simulink model "PI_real_expe"  (R2018a)
settings: Solver=FixedStepAuto  StartTime=0.0  StopTime=40  RelTol=1e-3
PreLoadFcn:
  | % plant
  | K0=0.82;
  | tau0=0.26;
  | 
  | % Sampling time
  | Ts=0.01;
  | 
  | % Especifications
  | xi=1;
  | ts_2=0.8; % settling time with %2 criterion
  | Tdes=ts_2/4;
  | wn=5.8/(xi*ts_2);
  | 
  | % Controller design
  | Zdes=exp(-Ts/Tdes);
  | alpha=exp(-Ts/tau0);
  | beta=-2*exp(-Ts*xi*wn)*cos(wn*Ts*sqrt(1-xi^2));
  | gamma=exp(-2*Ts*xi*wn);
  | 
  | Ki_star=(gamma-alpha+beta+(alpha+1))/(2*K0*(1-alpha));
  | Ki=(2/Ts)*Ki_star;
  | Kp=((beta+alpha+1)/(K0*(1-alpha)))-Ki_star;
undefined symbols (not defined in the file or in its folder): DiscIntNeverNeededParam
libraries: arduinolib x4, simulink x1
settings Model: SimulationMode=external  ExtModeTrigDuration=2  Creator=Eneko Lerma  LastModifiedBy=Eneko Lerma
settings OptimizationCC: EnhancedBackFolding=on  PassReuseOutputArgsAs=Individual arguments  MaxStackSize=64  OptimizeBlockOrder=speed  DifferentSizesBufferReuse=on  OptimizationCustomize=off
settings DebuggingCC: ParameterPrecisionLossMsg=none  ParameterTunabilityLossMsg=error
settings HardwareCC: ProdBitPerPointer=32  ProdBitPerSizeT=32  ProdBitPerPtrDiffT=32  ProdLargestAtomicInteger=Long  ProdLargestAtomicFloat=Double  ProdWordSize=32  ProdHWDeviceType=ARM Compatible->ARM Cortex
settings SFSimCC: MATLABDynamicMemAlloc=off
settings RTWCC: SystemTargetFile=ert.tlc  HardwareBoard=Arduino Due  TLCOptions=-aInlineSetEventsForThisBaseRateFcn=TLC_FALSE -aSuppressMultiTaskScheduler=TLC_FALSE -aRateBasedStepFcn=1  TemplateMakefile=ert_default_tmf  GenerateReport=on  Toolchain=Arduino ARM  BuildConfiguration=Faster Runs  IncludeHyperlinkInReport=on  LaunchReport=on  GenerateTraceInfo=on  GenerateTraceReport=on  GenerateTraceReportSl=on  GenerateTraceReportSf=on  GenerateTraceReportEml=on
settings RTWCC: CustomTerminator=|
  | writeDigitalPin((uint8_T)3, 0);
  | writeDigitalPin((uint8_T)5, 0);
settings CodeAppCC: ForceParamTrailComments=on  IgnoreCustomStorageClasses=off  OperatorAnnotations=on  SimulinkDataObjDesc=on  SFDataObjDesc=on  InsertBlockDesc=on
settings ERTTargetCC: SupportContinuousTime=on  SupportVariableSizeSignals=on

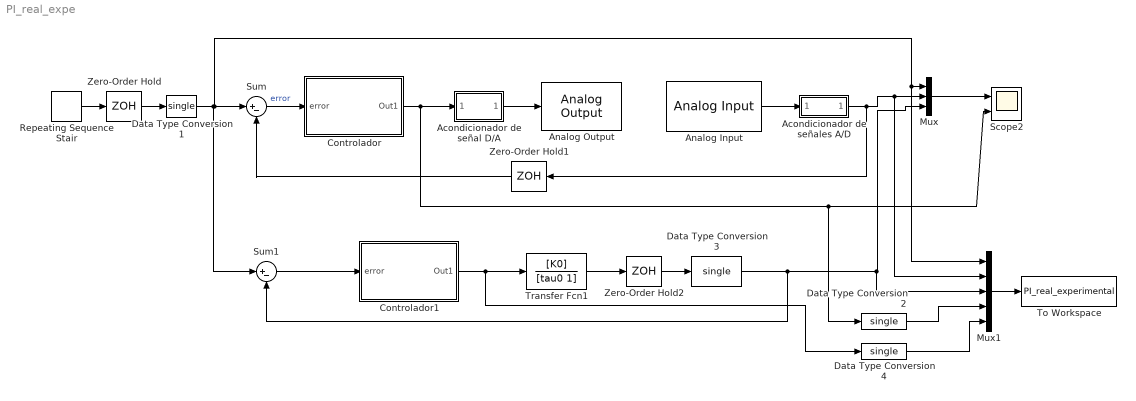
== system PI_real_expe ==
  Acondicionador de señal D/A : Subsystem
  Acondicionador de señales A/D : Subsystem
  Analog Input : arduinolib/Analog Input  pinNumber=0  ReadResultsOnly=off  ConversionTriggerSource=Software  ExternalTriggerType=uint32(0)  OutputDataType=uint16  EnableConversionCompleteNotify=off  EnableOuputStatus=off  SampleTime=0.005  blockPlatform=arduino
  Analog Output : arduinolib/Analog Output  DACpin=DAC1  blockPlatform=arduino
      settings: SourceProductName=Simulink Support Package for Arduino Hardware  SourceProductBaseCode=ARDUINO
  Controlador : Subsystem
  Controlador1 : Subsystem
  Data Type Conversion{1..4} (4 alike) : DataTypeConversion  OutDataTypeStr=single
  Mux : Mux  Inputs=3
  Mux1 : Mux  Inputs=5
  Repeating Sequence Stair : simulink/Sources/Repeating Sequence Stair  OutValues=[0 2 -2 -1].'  tsamp=4  OutMin=[]  OutMax=[]  OutDataTypeStr=double  OutputDataTypeScalingMode=double  OutDataType=fixdt(0,8)  ConRadixGroup=Best Precision: Vector-wise  OutScaling=2^-12
  Scope2 : Scope  NumInputPorts=2
  Sum : Sum  Inputs=|+-  AccumDataTypeStr=single
  Sum1 : Sum  Inputs=|+-  AccumDataTypeStr=single
  To Workspace : ToWorkspace  VariableName=PI_real_experimental  SaveFormat=Structure With Time  SampleTime=-1
  Transfer Fcn1 : TransferFcn  Numerator=[K0]  Denominator=[tau0 1]
  Zero-Order Hold : ZeroOrderHold  SampleTime=Ts
  Zero-Order Hold1 : ZeroOrderHold  SampleTime=Ts
  Zero-Order Hold2 : ZeroOrderHold  SampleTime=Ts
  wires:
  Mux/1 -> Scope2/1
  Acondicionador de señales A/D/1(" ") -> Mux1/2, Mux/2, Zero-Order Hold1/1
  Data Type Conversion1/1 -> Sum1/1, Sum/1, Mux1/1, Mux/1
  Sum/1 -> Controlador/1(error)  "error"
  Acondicionador de señal D/A/1(" ") -> Analog Output/1
  Analog Input/1 -> Acondicionador de señales A/D/1("  ")
  Controlador/1(Out1) -> Data Type Conversion2/1, Scope2/2, Acondicionador de señal D/A/1("  ")
  Zero-Order Hold/1 -> Data Type Conversion1/1
  Zero-Order Hold1/1 -> Sum/2
  Controlador1/1(Out1) -> Data Type Conversion4/1, Transfer Fcn1/1
  Sum1/1 -> Controlador1/1(error)
  Transfer Fcn1/1 -> Zero-Order Hold2/1
  Zero-Order Hold2/1 -> Data Type Conversion3/1
  Data Type Conversion3/1 -> Sum1/2, Mux1/3, Mux/3
  Repeating Sequence Stair/1 -> Zero-Order Hold/1
  Mux1/1 -> To Workspace/1
  Data Type Conversion2/1 -> Mux1/4
  Data Type Conversion4/1 -> Mux1/5

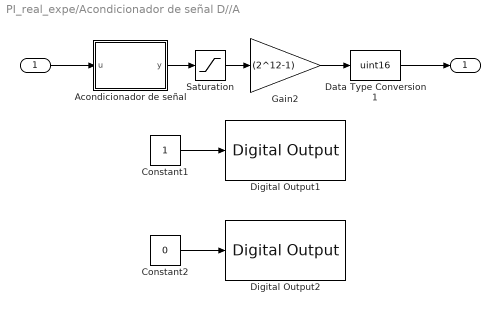
== system PI_real_expe/Acondicionador de señal D//A ==
  "  " : Inport  OutDataTypeStr=double
  Acondicionador de señal : MATLAB Function  TreatAsAtomicUnit=on
  Constant1 : Constant
  Constant2 : Constant  Value=0
  Data Type Conversion1 : DataTypeConversion  OutDataTypeStr=uint16
  Digital Output1 : arduinolib/Digital Output  pinNumber=5  blockPlatform=arduino
  Digital Output2 : arduinolib/Digital Output  pinNumber=3  blockPlatform=arduino
  Gain2 : Gain  Gain=(2^12-1)  OutDataTypeStr=single
  Saturation : Saturate  UpperLimit=1  LowerLimit=0  OutDataTypeStr=single
  " " : Outport  OutDataTypeStr=uint16
  wires:
  Gain2/1 -> Data Type Conversion1/1
  "  "/1 -> Acondicionador de señal/1(u)
  Acondicionador de señal/1(y) -> Saturation/1
  Data Type Conversion1/1 -> " "/1
  Saturation/1 -> Gain2/1
  Constant1/1 -> Digital Output1/1
  Constant2/1 -> Digital Output2/1

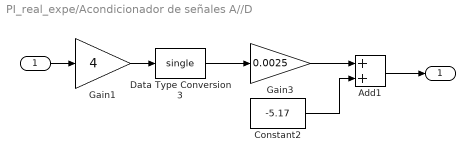
== system PI_real_expe/Acondicionador de señales A//D ==
  "  " : Inport  OutDataTypeStr=uint16
  Add1 : Sum  AccumDataTypeStr=single
  Constant2 : Constant  Value=-5.17  OutDataTypeStr=single
  Data Type Conversion3 : DataTypeConversion  OutDataTypeStr=single
  Gain1 : Gain  Gain=4  OutDataTypeStr=uint16
  Gain3 : Gain  Gain=0.0025  OutDataTypeStr=single
  " " : Outport  OutDataTypeStr=single
  wires:
  Gain1/1 -> Data Type Conversion3/1
  "  "/1 -> Gain1/1
  Data Type Conversion3/1 -> Gain3/1
  Gain3/1 -> Add1/1
  Constant2/1 -> Add1/2
  Add1/1 -> " "/1

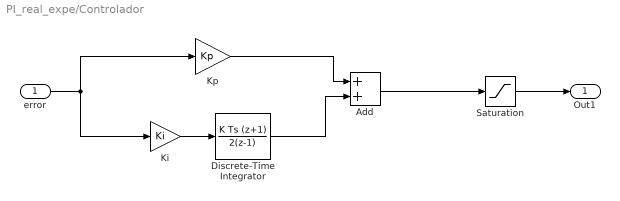
== system PI_real_expe/Controlador ==
  error : Inport
  Add : Sum  AccumDataTypeStr=single
  Discrete-Time Integrator : DiscreteIntegrator  IntegratorMethod=Integration: Trapezoidal  SampleTime=Ts  OutDataTypeStr=single  ICPrevOutput=DiscIntNeverNeededParam  ICPrevScaledInput=DiscIntNeverNeededParam
  Ki : Gain  Gain=Ki
  Kp : Gain  Gain=Kp  OutDataTypeStr=single
  Saturation : Saturate  UpperLimit=5  LowerLimit=-5  OutDataTypeStr=double
  Out1 : Outport  OutDataTypeStr=double
  wires:
  Kp/1 -> Add/1
  Discrete-Time Integrator/1 -> Add/2
  Ki/1 -> Discrete-Time Integrator/1
  Add/1 -> Saturation/1
  Saturation/1 -> Out1/1
  error/1 -> Ki/1, Kp/1

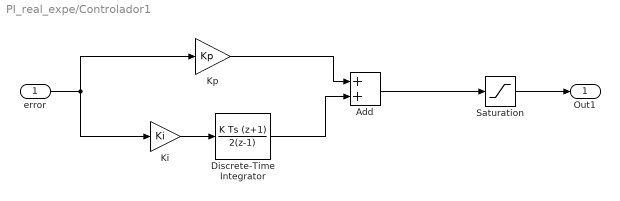
== system PI_real_expe/Controlador1 ==
  error : Inport
  Add : Sum  AccumDataTypeStr=single
  Discrete-Time Integrator : DiscreteIntegrator  IntegratorMethod=Integration: Trapezoidal  SampleTime=Ts  OutDataTypeStr=single  ICPrevOutput=DiscIntNeverNeededParam  ICPrevScaledInput=DiscIntNeverNeededParam
  Ki : Gain  Gain=Ki
  Kp : Gain  Gain=Kp  OutDataTypeStr=single
  Saturation : Saturate  UpperLimit=5  LowerLimit=-5  OutDataTypeStr=double
  Out1 : Outport  OutDataTypeStr=double
  wires:
  error/1 -> Kp/1, Ki/1
  Saturation/1 -> Out1/1
  Add/1 -> Saturation/1
  Ki/1 -> Discrete-Time Integrator/1
  Discrete-Time Integrator/1 -> Add/2
  Kp/1 -> Add/1

== matlab function PI_real_expe/Acondicionador de señal D//A/Acondicionador de señal ==
  data: u input; y output
function y = fcn(u)
y =0.0961*u+0.5099;
